simulink model "PAmmodem"  (R2016a)
settings: Solver=VariableStepDiscrete  StartTime=0.0  StopTime=100  RelTol=1e-3
libraries: commdigbbndam3 x2, simulink_extras x2, commchan3 x1, commsink2 x1, commrandsrc3 x1
settings Model: Creator=medo_  LastModifiedBy=medo_

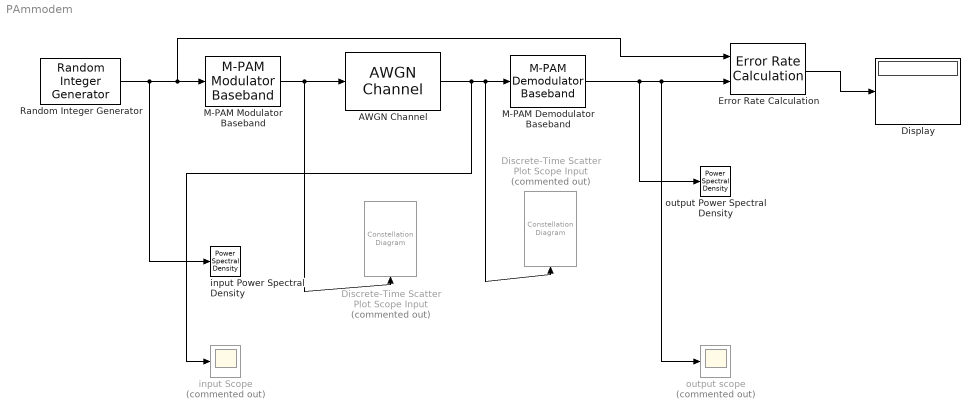
== system PAmmodem ==
  AWGN Channel : commchan3/AWGN Channel  InputProcessing=Columns as channels (frame based)  seed=37  noiseMode="Signal to noise ratio  (SNR)"  EbNodB=10  EsNodB=10  SNRdB=10  bitsPerSym=1  Ps=1  Tsym=0.1  variance=1
  Discrete-Time Scatter Plot Scope Input : ConstellationDiagram  Tag=ScatterPlot  Commented=on
  "Discrete-Time Scatter Plot Scope Input " : ConstellationDiagram  Tag=ScatterPlot  Commented=on
  Display : Display
  Error Rate Calculation : commsink2/Error Rate Calculation  N=0  st_delay=0  cp_mode=Entire frame  subframe=[]  PMode=Port  WsName=ErrorVec  RsMode2=off  stop=off  numErr=100  maxBits=1e6
  M-PAM Demodulator Baseband : commdigbbndam3/M-PAM Demodulator Baseband  M=4  OutType=Integer  Dec=Binary  PowType=Peak Power  MinDist=2  AvgPow=1  PeakPow=1  outDtype1=Inherit via internal rule  outDtype2=Inherit via internal rule  denormFactorWordLen=16  denormFactorDataTypeStr=Inherit: Same word length as input  denormFactorLastDataTypeStr=Inherit: Same word length as input  prodOutWordLen=16  prodOutRoundingMode=Floor  prodOutOverflowMode=Wrap  prodOutOvFlMode=off  prodOutOvFlModeLastStrValue=off  sumWordLen=16
  M-PAM Modulator Baseband : commdigbbndam3/M-PAM Modulator Baseband  M=4  InType=Integer  Enc=Binary  PowType=Peak Power  MinDist=2  AvgPow=1  PeakPow=1  outDtype=double  outWordLen=16  outUDDataType=sfix(16)  outFracLenMode=Best precision  outFracLen=15  outDataTypeStr=double  outLastDataTypeStr=double
  Random Integer Generator : commrandsrc3/Random Integer Generator  SetSize=4  SeedSource=Auto  Seed=0  SampleTime=0.1  SamplesPerFrame=1  OutputDataType=double  SimulateUsing=Interpreted execution
  input Scope : Scope  Commented=on
  input Power Spectral Density : simulink_extras/Additional Sinks/Power Spectral Density  npts=128  fftpts=512  HowOften=64  sampleT=0.1
  output Power Spectral Density : simulink_extras/Additional Sinks/Power Spectral Density  npts=128  fftpts=512  HowOften=64  sampleT=0.1
  output scope : Scope  Commented=on
  wires:
  M-PAM Modulator Baseband/1 -> Discrete-Time Scatter Plot Scope Input/1, AWGN Channel/1
  M-PAM Demodulator Baseband/1 -> output scope/1, Error Rate Calculation/2, output Power Spectral Density/1
  Random Integer Generator/1 -> input Power Spectral Density/1, Error Rate Calculation/1, M-PAM Modulator Baseband/1
  AWGN Channel/1 -> input Scope/1, "Discrete-Time Scatter Plot Scope Input "/1, M-PAM Demodulator Baseband/1
  Error Rate Calculation/1 -> Display/1
